simulink model "PosFBGenerator_with_PCNN_simulator"  (Simulink 8.4)
settings: Solver=ode45  StartTime=0.0  StopTime=6  RelTol=1e-3
libraries: NeuroModelerLibrary x7
settings Model: Creator=Bakhshiev  LastModifiedBy=Tim

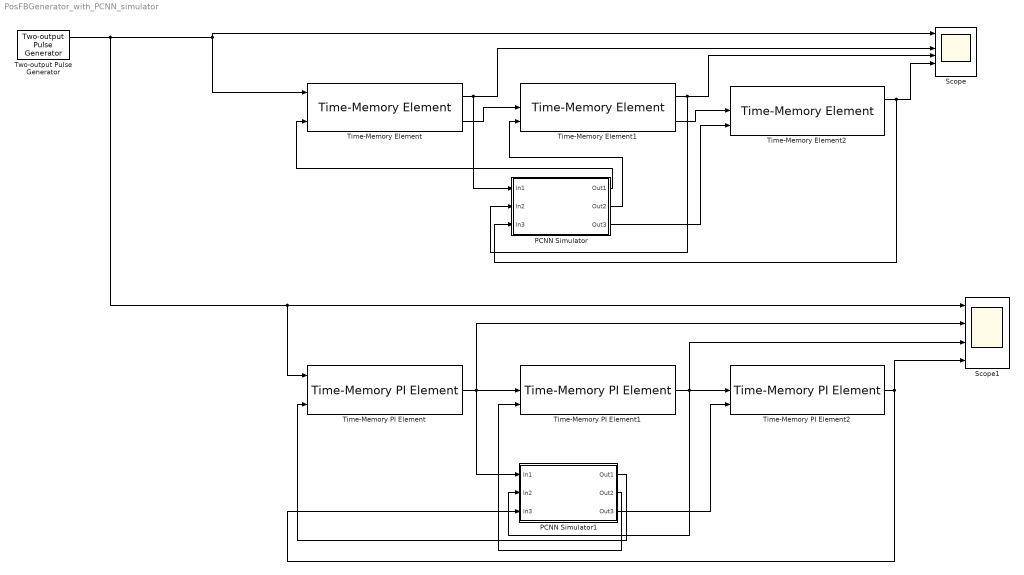
== system PosFBGenerator_with_PCNN_simulator ==
  PCNN Simulator : Subsystem  mask{TimeDelay=1, NumIOs=5}
      mask prompts: TimeDelay "Enter Time Delay"; NumIOs "Enter Num IOs"
  PCNN Simulator1 : Subsystem  mask{TimeDelay=0.1, NumIOs=5}
      mask prompts: TimeDelay "Enter Time Delay"; NumIOs "Enter Num IOs"
  Scope : Scope  NumInputPorts=6
      settings: YMin=0~-1~0~0~0~-1  YMax=1~1~1~1~1~1  MaxDataPoints=500000
  Scope1 : Scope  NumInputPorts=4
      settings: YMin=0~-1~0~0  YMax=1~1~1~1  MaxDataPoints=500000
  Time-Memory Element : NeuroModelerLibrary/Memory Modules/Time-Memory Element
  Time-Memory Element1 : NeuroModelerLibrary/Memory Modules/Time-Memory Element
  Time-Memory Element2 : NeuroModelerLibrary/Memory Modules/Time-Memory Element
  Time-Memory PI Element : NeuroModelerLibrary/Memory Modules/Time-Memory PI Element
  Time-Memory PI Element1 : NeuroModelerLibrary/Memory Modules/Time-Memory PI Element
  Time-Memory PI Element2 : NeuroModelerLibrary/Memory Modules/Time-Memory PI Element
  Two-output Pulse Generator : NeuroModelerLibrary/Support/Two-output Pulse Generator  A=1  P1=10000  P2=30  PW=1  ST=0.001  OOn1=2  OOff1=7700  OOn2=0  OOff2=7000
  wires:
  Two-output Pulse Generator/1 -> Time-Memory PI Element/1, Scope1/1, Time-Memory Element/1, Scope/1
  Time-Memory Element/1 -> PCNN Simulator/1(In1), Scope/3
  Time-Memory Element/2 -> Time-Memory Element1/2
  Time-Memory Element1/2 -> Time-Memory Element2/2
  Time-Memory Element1/1 -> PCNN Simulator/2(In2), Scope/4
  Time-Memory Element2/1 -> PCNN Simulator/3(In3), Scope/5
  PCNN Simulator/1(Out1) -> Time-Memory Element/3
  PCNN Simulator/2(Out2) -> Time-Memory Element1/3
  PCNN Simulator/3(Out3) -> Time-Memory Element2/3
  Time-Memory PI Element/1 -> Scope1/2, PCNN Simulator1/1(In1), Time-Memory PI Element1/2
  Time-Memory PI Element1/1 -> Scope1/3, PCNN Simulator1/2(In2), Time-Memory PI Element2/2
  PCNN Simulator1/1(Out1) -> Time-Memory PI Element/3
  PCNN Simulator1/2(Out2) -> Time-Memory PI Element1/3
  Time-Memory PI Element2/1 -> Scope1/4, PCNN Simulator1/3(In3)
  PCNN Simulator1/3(Out3) -> Time-Memory PI Element2/3

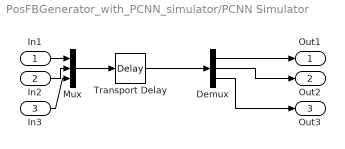
== system PosFBGenerator_with_PCNN_simulator/PCNN Simulator ==
  In1 : Inport
  In2 : Inport  Port=2
  In3 : Inport  Port=3
  Demux : Demux  Outputs=3
  Mux : Mux  Inputs=3
  Transport Delay : TransportDelay  DelayTime=TimeDelay
  Out1 : Outport
  Out2 : Outport  Port=2
  Out3 : Outport  Port=3
  wires:
  Demux/2 -> Out2/1
  In1/1 -> Mux/1
  In2/1 -> Mux/2
  Demux/1 -> Out1/1
  Transport Delay/1 -> Demux/1
  Mux/1 -> Transport Delay/1
  In3/1 -> Mux/3
  Demux/3 -> Out3/1

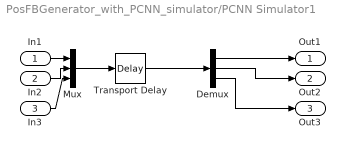
== system PosFBGenerator_with_PCNN_simulator/PCNN Simulator1 ==
  In1 : Inport
  In2 : Inport  Port=2
  In3 : Inport  Port=3
  Demux : Demux  Outputs=3
  Mux : Mux  Inputs=3
  Transport Delay : TransportDelay  DelayTime=TimeDelay
  Out1 : Outport
  Out2 : Outport  Port=2
  Out3 : Outport  Port=3
  wires:
  Demux/2 -> Out2/1
  In1/1 -> Mux/1
  In2/1 -> Mux/2
  Demux/1 -> Out1/1
  Transport Delay/1 -> Demux/1
  Mux/1 -> Transport Delay/1
  In3/1 -> Mux/3
  Demux/3 -> Out3/1
